simulink model "ckhsigselftestsigtest01"  (R2016a)
settings: Solver=VariableStepAuto  StartTime=0.0  StopTime=10.0  RelTol=1e-3
libraries: dspsrcs4 x1
settings Model: Creator=khung  LastModifiedBy=khung
settings DebuggingCC: SolverPrmCheckMsg=warning  AllowSymbolicDim=off
settings ModelReferenceCC: PropagateSignalLabelsOutOfModel=off
settings ConfigComp: CovModelRefEnable=Off  CovSFcnEnable=off

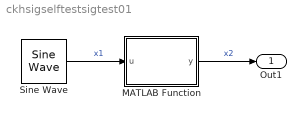
== system ckhsigselftestsigtest01 ==
  MATLAB Function : MATLAB Function  TreatAsAtomicUnit=on
  Sine Wave : dspsrcs4/Sine Wave  Amplitude=1  Frequency=100  Phase=0  SampleMode=Discrete  OutComplex=Real  CompMethod=Trigonometric fcn  TableSize=Speed  SampleTime=1  SamplesPerFrame=1  ResetState=Restart at time zero  OutputFrames=off  dataType=double  wordLen=16  udDataType=sfix(16)  fracBitsMode=Best precision  numFracBits=15  OutDataTypeStr=double  LastOutDataTypeStr=double
  Out1 : Outport
  wires:
  Sine Wave/1 -> MATLAB Function/1(u)  "x1"
  MATLAB Function/1(y) -> Out1/1  "x2"

== matlab function ckhsigselftestsigtest01/MATLAB Function ==
  data: u input; y output
function y = fcn(u)
%#codegen

y = u;
% size(y)
